simulink library "MyLib"  (R2024b)
settings: Solver=VariableStepAuto  StartTime=0.0  StopTime=10.0  RelTol=1e-3
libraries: spsIGBTDiodeLib x4, spsSeriesRLCBranchLib x2, simulink x1, spsDCVoltageSourceLib x1, spsVoltageMeasurementLib x1
settings Model: Creator=tiany  LastModifiedBy=tiany

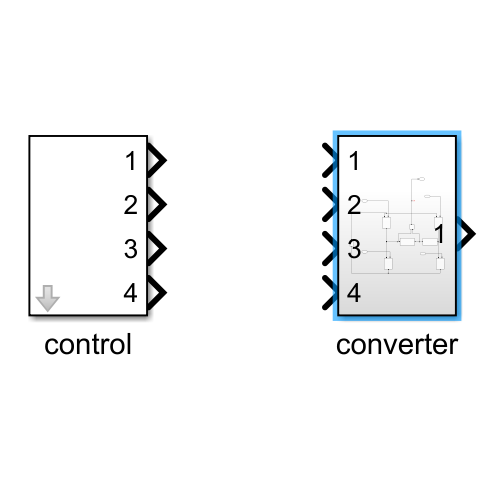
[thumbnail: Simulink's stored preview of the top-level diagram]
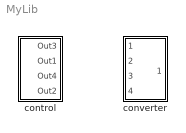
== system MyLib ==
  control : Subsystem  mask{Repeating_Sequence_rep_seq_y=[-1, 0, -1], SineWave_Amplitude=1, SineWave_Bias=0, SineWave_Frequency=100*pi, SineWave_Phase=0}
      mask prompts: Repeating_Sequence_rep_seq_y "Repeating Sequence.rep_seq_y"; SineWave_Amplitude "Sine Wave.Amplitude"; SineWave_Bias "Sine Wave.Bias"; SineWave_Frequency "Sine Wave.Frequency"; SineWave_Phase "Sine Wave.Phase"
      mask DialogControl DescTextVar Prompt: 桥式逆变控制回路
      mask DialogControl ParameterGroupVar Prompt: paramerters
  converter : Subsystem

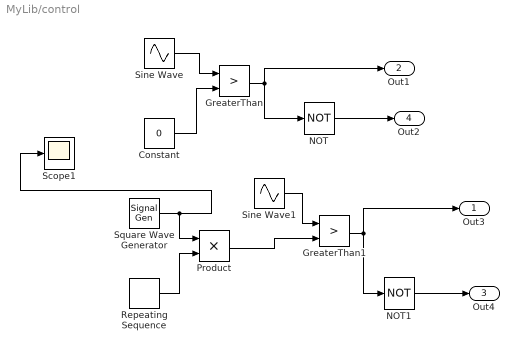
== system MyLib/control ==
  Constant : Constant  Value=0
  GreaterThan : RelationalOperator  Operator=>  OutDataTypeStr=boolean  RndMeth=Simplest  InputSameDT=off
  GreaterThan1 : RelationalOperator  Operator=>  OutDataTypeStr=boolean  RndMeth=Simplest  InputSameDT=off
  NOT : Logic  Operator=NOT  IconShape=distinctive  AllPortsSameDT=off  OutDataTypeStr=boolean
  NOT1 : Logic  Operator=NOT  IconShape=distinctive  AllPortsSameDT=off  OutDataTypeStr=boolean
  Product : Product
  Repeating Sequence : simulink/Sources/Repeating Sequence  rep_seq_t=[0, 1/10000/2, 1/10000]  rep_seq_y=Repeating_Sequence_rep_seq_y
  Scope1 : Scope
  Sine Wave : Sin  Amplitude=SineWave_Amplitude  Bias=SineWave_Bias  Frequency=SineWave_Frequency  Phase=SineWave_Phase  SampleTime=0
  Sine Wave1 : Sin  Frequency=100*pi  SampleTime=0
  Square Wave Generator : SignalGenerator  WaveForm=square  Frequency=50
  Out3 : Outport
  Out1 : Outport  Port=2
  Out4 : Outport  Port=3
  Out2 : Outport  Port=4
  wires:
  GreaterThan1/1 -> Out3/1, NOT1/1
  Sine Wave1/1 -> GreaterThan1/1
  Square Wave Generator/1 -> Scope1/1, Product/1
  GreaterThan/1 -> Out1/1, NOT/1
  Sine Wave/1 -> GreaterThan/1
  Repeating Sequence/1 -> Product/2
  Product/1 -> GreaterThan1/2
  Constant/1 -> GreaterThan/2
  NOT1/1 -> Out4/1
  NOT/1 -> Out2/1

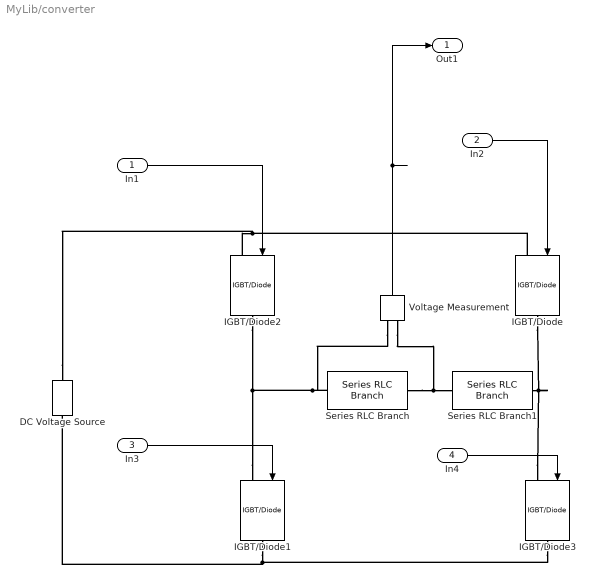
== system MyLib/converter ==
  In1 : Inport
  In2 : Inport  Port=2
  In3 : Inport  Port=3
  In4 : Inport  Port=4
  DC Voltage Source : spsDCVoltageSourceLib/DC Voltage Source  Amplitude=100  Measurements=Voltage
  IGBT/Diode{,1..3} (4 alike) : spsIGBTDiodeLib/IGBT//Diode  Ron=1e-3  Rs=1e5  Cs=inf  Measurements=off
  Series RLC Branch : spsSeriesRLCBranchLib/Series RLC Branch  LConnTagsString=__new0  RConnTagsString=__new0  BranchType=R  Resistance=10  Inductance=1e-3  SetiL0=off  InitialCurrent=0  Capacitance=1e-6  Setx0=off  InitialVoltage=0  Measurements=None
  Series RLC Branch1 : spsSeriesRLCBranchLib/Series RLC Branch  LConnTagsString=__new0  RConnTagsString=__new0  BranchType=L  Resistance=10  Inductance=0.001  SetiL0=off  InitialCurrent=0  Capacitance=1e-6  Setx0=off  InitialVoltage=0  Measurements=None
  Voltage Measurement : spsVoltageMeasurementLib/Voltage Measurement  PhasorSimulation=off  OutputType=Complex  PSBequivalent=0
  Out1 : Outport
  wires:
  Voltage Measurement/1 -> Out1/1
  In1/1 -> IGBT/Diode2/1
  In2/1 -> IGBT/Diode/1
  In3/1 -> IGBT/Diode1/1
  In4/1 -> IGBT/Diode3/1
  connections:
  DC Voltage Source/RConn1 -- IGBT/Diode2/LConn1 -- IGBT/Diode/LConn1
  Voltage Measurement/LConn2 -- Series RLC Branch/RConn1 -- Series RLC Branch1/LConn1
  IGBT/Diode3/LConn1 -- Series RLC Branch1/RConn1 -- IGBT/Diode/RConn1
  IGBT/Diode1/LConn1 -- IGBT/Diode2/RConn1 -- Voltage Measurement/LConn1 -- Series RLC Branch/LConn1
  DC Voltage Source/LConn1 -- IGBT/Diode1/RConn1 -- IGBT/Diode3/RConn1
